simulink model "simu5"  (R2018b)
settings: Solver=FixedStepAuto  StartTime=0.0  StopTime=10.0  FixedStep=0.01  MinStep=0.2  RelTol=1e-3
values from neighbouring files (symbols this model uses):
  du = 1    [script5.m]
  ksi = 1/(i+1)    [script5.m]
  omega = 1/ksi    (= 4)    [script5.m]
  t0 = 0    [script5.m]
  u0 = 0    [script5.m]
settings Model: Creator=wojciechkonury  LastModifiedBy=wojciechkonury

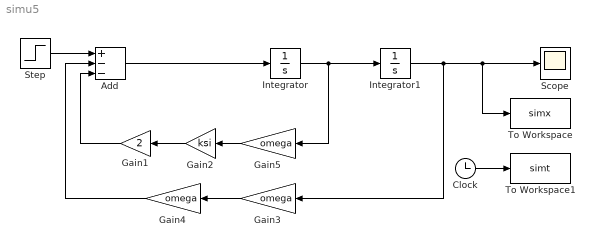
== system simu5 ==
  Add : Sum  Inputs=+--
  Clock : Clock
  Gain1 : Gain  Gain=2
  Gain2 : Gain  Gain=ksi
  Gain3 : Gain  Gain=omega
  Gain4 : Gain  Gain=omega
  Gain5 : Gain  Gain=omega
  Integrator : Integrator
  Integrator1 : Integrator
  Scope : Scope
  Step : Step  Time=t0  Before=u0  After=u0 + du  SampleTime=0
  To Workspace : ToWorkspace  VariableName=simx  SampleTime=-1
      settings: Save2DSignal=2-D array (concatenate along first dimension)
  To Workspace1 : ToWorkspace  VariableName=simt  SampleTime=-1
      settings: Save2DSignal=2-D array (concatenate along first dimension)
  wires:
  Add/1 -> Integrator/1
  Integrator/1 -> Gain5/1, Integrator1/1
  Gain1/1 -> Add/3
  Integrator1/1 -> Gain3/1, To Workspace/1, Scope/1
  Step/1 -> Add/1
  Clock/1 -> To Workspace1/1
  Gain2/1 -> Gain1/1
  Gain5/1 -> Gain2/1
  Gain3/1 -> Gain4/1
  Gain4/1 -> Add/2
